simulink model "Simple_Pendulum_Motion"  (R2024a)
settings: Solver=FixedStepAuto  StartTime=0.0  StopTime=10.0  FixedStep=1E-3  RelTol=1e-3
values from neighbouring files (symbols this model uses):
  g = 9.81    [Simple_Pendulum.m]
  L = 0.001    [Simple_Pendulum.m]
settings Model: Creator=VICTUS  LastModifiedBy=VICTUS

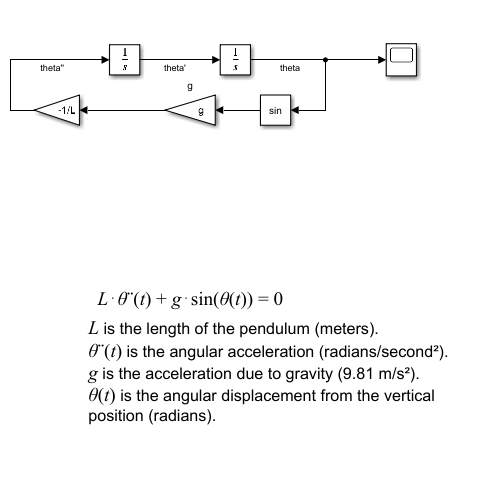
[thumbnail: Simulink's stored preview of the top-level diagram]
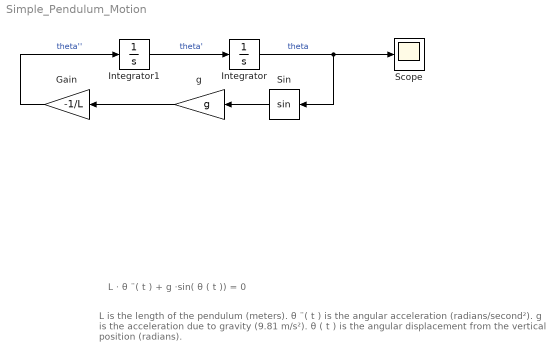
== system Simple_Pendulum_Motion ==
  note: L ⋅ θ ¨( t ) + g ⋅sin( θ ( t )) = 0
  note: L is the length of the pendulum (meters).
      | θ ¨( t ) is the angular acceleration (radians/second²).
      | g is the acceleration due to gravity (9.81 m/s²).
      | θ ( t ) is the angular displacement from the vertical position (radians).
  Gain : Gain  Gain=-1/L
  Integrator : Integrator  InitialCondition=1
  Integrator1 : Integrator
  Scope : Scope
  Sin : Trigonometry  OutputSignalType=real
  g : Gain  Gain=g
  wires:
  Integrator1/1 -> Integrator/1  "theta'"
  Gain/1 -> Integrator1/1  "theta''"
  Integrator/1 -> Scope/1, Sin/1  "theta"
  Sin/1 -> g/1
  g/1 -> Gain/1
